simulink model "pmsm_plant"  (R2024b)
settings: Solver=VariableStepAuto  StartTime=0.0  StopTime=10.0  RelTol=1e-3
values from neighbouring files (symbols this model uses):
  J = 0.01    [step5a_plant.m]    (also in step5b_current_control.m; step5c_speed_control.m; step5d_position_control.m)
  Ld_nom = 0.001    [step5a_plant.m]    (also in step5b_current_control.m; step5c_speed_control.m; step5d_position_control.m)
  Lq_nom = 0.001    [step5a_plant.m]    (also in step5b_current_control.m; step5c_speed_control.m; step5d_position_control.m)
  PolePairs = 3    [step5a_plant.m]    (also in step5b_current_control.m; step5c_speed_control.m; step5d_position_control.m)
  psi_d_nom = 0.08    [step5a_plant.m]    (also in step5b_current_control.m; step5c_speed_control.m; step5d_position_control.m)
  Rs = interp1(obj.TempGrid, obj.RsMap, temperature, 'linear', 'extrap')    [SurfaceMountedPMSM.m]    (also in simulate_surface_pmsm_foc.m = motor.interpRs(temperature); step1_build_plant_openloop.m = motor.interpRs(temperature); step2_build_current_loop_svpwm.m = motor.interpRs(temperature); step3_build_speed_loop.m = motor.interpRs(temperature))
settings Model: Creator=Lee  LastModifiedBy=Lee

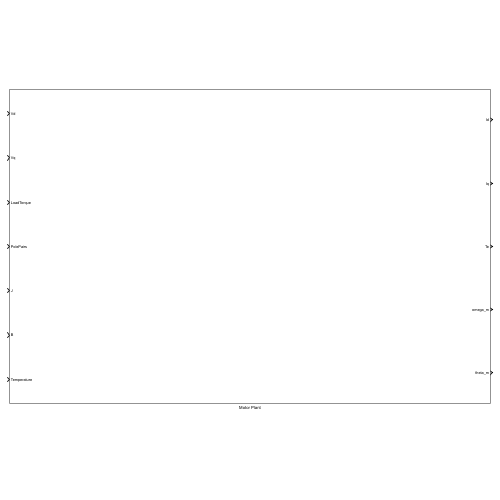
[thumbnail: Simulink's stored preview of the top-level diagram]
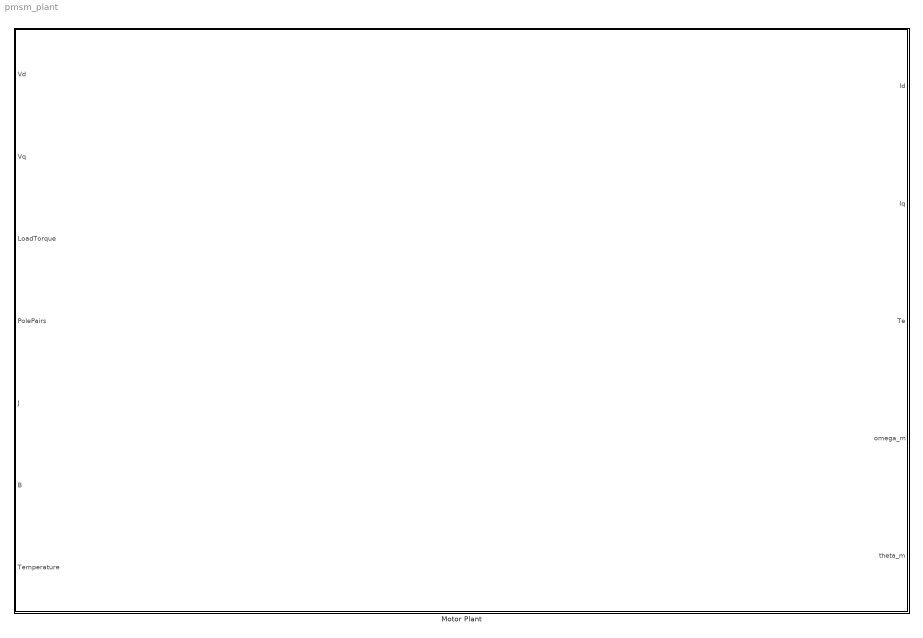
== system pmsm_plant ==
  Motor Plant : Subsystem

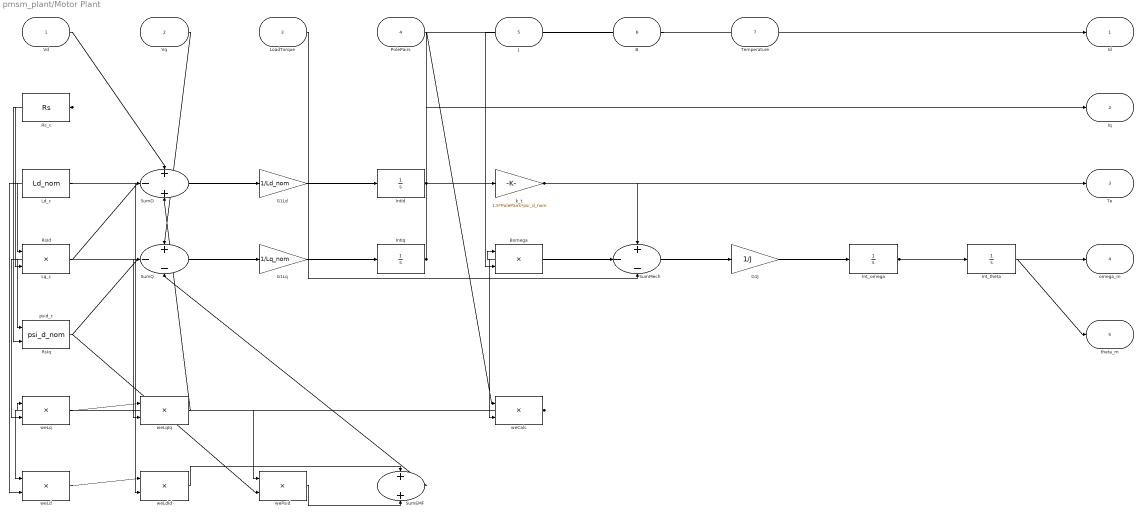
== system pmsm_plant/Motor Plant ==
  Vd : Inport
  Vq : Inport  Port=2
  LoadTorque : Inport  Port=3
  PolePairs : Inport  Port=4
  J : Inport  Port=5
  B : Inport  Port=6
  Temperature : Inport  Port=7
  Bomega : Product
  G1J : Gain  Gain=1/J
  G1Ld : Gain  Gain=1/Ld_nom
  G1Lq : Gain  Gain=1/Lq_nom
  IntId : Integrator
  IntIq : Integrator
  Int_omega : Integrator
  Int_theta : Integrator
  Ld_c : Constant  Value=Ld_nom
  Lq_c : Constant  Value=Lq_nom
  RsId : Product
  RsIq : Product
  Rs_c : Constant  Value=Rs
  SumD : Sum  Inputs=+-+
  SumEMF : Sum
  SumMech : Sum  Inputs=+--
  SumQ : Sum  Inputs=+--
  k_t : Gain  Gain=1.5*PolePairs*psi_d_nom
  psid_c : Constant  Value=psi_d_nom
  weCalc : Product
  weLd : Product
  weLdId : Product
  weLq : Product
  weLqIq : Product
  wePsid : Product
  Id : Outport
  Iq : Outport  Port=2
  Te : Outport  Port=3
  omega_m : Outport  Port=4
  theta_m : Outport  Port=5
  wires:
  ? -> ?
  Vd/1 -> SumD/1
  IntId/1 -> RsId/1, Id/1, weLdId/2
  Rs_c/1 -> RsId/2, RsIq/2
  RsId/1 -> SumD/2
  weLqIq/1 -> SumD/3
  SumD/1 -> G1Ld/1
  G1Ld/1 -> IntId/1
  Vq/1 -> SumQ/1
  IntIq/1 -> RsIq/1, Iq/1, weLqIq/2, k_t/1
  RsIq/1 -> SumQ/2
  SumEMF/1 -> SumQ/3
  SumQ/1 -> G1Lq/1
  G1Lq/1 -> IntIq/1
  PolePairs/1 -> weCalc/1
  Int_omega/1 -> weCalc/2, Bomega/1, Int_theta/1, omega_m/1
  weCalc/1 -> weLq/1, weLd/1, wePsid/1
  Lq_c/1 -> weLq/2
  weLq/1 -> weLqIq/1
  Ld_c/1 -> weLd/2
  weLd/1 -> weLdId/1
  psid_c/1 -> wePsid/2
  weLdId/1 -> SumEMF/1
  wePsid/1 -> SumEMF/2
  k_t/1 -> SumMech/1, Te/1
  B/1 -> Bomega/2
  Bomega/1 -> SumMech/2
  LoadTorque/1 -> SumMech/3
  SumMech/1 -> G1J/1
  G1J/1 -> Int_omega/1
  Int_theta/1 -> theta_m/1
